simulink library "Lib_Cntrl_FirstOrderActuator_TMATS"  (R2012b)
settings: Solver=ode45  StartTime=0.0  StopTime=10.0  RelTol=1e-3
Description:
  | Thomas Modules
settings Model: Creator=jwchapm2  LastModifiedBy=jwchapm2

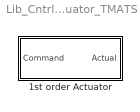
== system Lib_Cntrl_FirstOrderActuator_TMATS ==
  1st order Actuator : Subsystem  mask(T-MATS: 1st Order Actuator Library Block){Gain_M=1, Tau_M=0.01, IC_M=0, MaxSat_M=100, MinSat_M=0, deadband_M=0.05, rateLimit_M=2}
      mask prompts: Gain_M "Gain_M - Sensor Gain"; Tau_M "Tau_M - Sensor Time Constant"; IC_M "IC_M - Initial Condition"; MaxSat_M "MaxSat_M - Actuator Max Saturation point"; MinSat_M "MinSat_M - Actuator Min Saturation point"; deadband_M "deadband_M - Acturator deadband"; rateLimit_M "rateLimit_M - Acturator rate limit"
      mask help: This block models a generic actuator with a first order lag.
      mask Help: web(which('Control_TMATS_1OA.html'),'-helpbrowser')

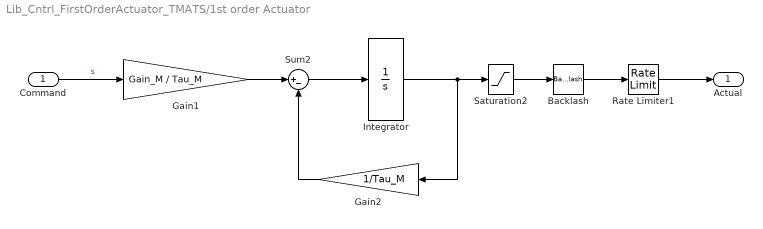
== system Lib_Cntrl_FirstOrderActuator_TMATS/1st order Actuator ==
  Command : Inport
  Backlash : Backlash  BacklashWidth=deadband_M  InitialOutput=IC_M
  Gain1 : Gain  Gain=Gain_M / Tau_M
  Gain2 : Gain  Gain=1/Tau_M
  Integrator : Integrator  InitialCondition=IC_M
  Rate Limiter1 : RateLimiter  RisingSlewLimit=rateLimit_M  FallingSlewLimit=-1*rateLimit_M  SampleTimeMode=inherited  InitialCondition=IC_M
  Saturation2 : Saturate  UpperLimit=MaxSat_M  LowerLimit=MinSat_M
  Sum2 : Sum  Inputs=|+-
  Actual : Outport
  wires:
  Backlash/1 -> Rate Limiter1/1
  Command/1 -> Gain1/1  "s"
  Rate Limiter1/1 -> Actual/1
  Gain1/1 -> Sum2/1
  Sum2/1 -> Integrator/1
  Gain2/1 -> Sum2/2
  Integrator/1 -> Gain2/1, Saturation2/1
  Saturation2/1 -> Backlash/1
